simulink model "Gastro_Insulin34"  (R2018a)
settings: Solver=VariableStepAuto  StartTime=0.0  StopTime=10.0  RelTol=1e-3
undefined symbols (not defined in the file): Q_i_G, V_i_G
settings Model: Creator=cgonterman  LastModifiedBy=cgonterman

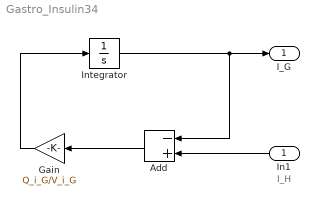
== system Gastro_Insulin34 ==
  note: I_H
  In1 : Inport
  Add : Sum  Inputs=-+
  Gain : Gain  Gain=Q_i_G/V_i_G
  Integrator : Integrator
  "I_G " : Outport
  wires:
  In1/1 -> Add/2
  Add/1 -> Gain/1
  Gain/1 -> Integrator/1
  Integrator/1 -> Add/1, "I_G "/1
